simulink model "rc"  (R2019a)
settings: Solver=VariableStepAuto  StartTime=0.0  StopTime=10.0  RelTol=1e-3
values from neighbouring files (symbols this model uses):
  C = 1E-6    (= 1e-06)    [CLab1.m]
  F = [2*pi*1, 2*pi*10, 2*pi*100]    [CLab1.m]
  R = 10000    [CLab1.m]
settings Model: Creator=Pranav Maddula  LastModifiedBy=Pranav Maddula

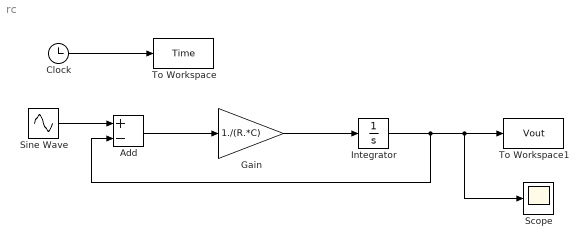
== system rc ==
  Add : Sum  Inputs=+-
  Clock : Clock
  Gain : Gain  Gain=1./(R.*C)
  Integrator : Integrator
  Scope : Scope
  Sine Wave : Sin  Frequency=F  SampleTime=0
  To Workspace : ToWorkspace  VariableName=Time  SampleTime=-1
  To Workspace1 : ToWorkspace  VariableName=Vout  SampleTime=-1
  wires:
  Clock/1 -> To Workspace/1
  Sine Wave/1 -> Add/1
  Add/1 -> Gain/1
  Gain/1 -> Integrator/1
  Integrator/1 -> Add/2, Scope/1, To Workspace1/1
